simulink model "Acceleration"  (R2017a)
settings: Solver=VariableStepAuto  StartTime=0.0  StopTime=5  FixedStep=0.0001  RelTol=1e-3
values from neighbouring files (symbols this model uses):
  Fz0 = 450*g    (= 4414.5)    [variabeln.m]
  g = 9.81    [variabeln.m]
  gear_ratio = 7.13    [variabeln.m]
  h_CoM = 0.5    [variabeln.m]
  J = 1    [variabeln.m]
  K_i = 100    [variabeln.m]
  l = l_f+l_r    (= 3)    [variabeln.m]
  l_f = 1.5    [variabeln.m]
  lambda_target = 0.1    [variabeln.m]
  m = 700    [variabeln.m]
  max_torque = 220    [variabeln.m]
  Q = 1000    [variabeln.m]
  R = 0.01    [variabeln.m]
  r = 0.25    [variabeln.m]
  Ta0 = 800    [variabeln.m]
  theta1 = 0.86    [variabeln.m]
  theta2 = 33.82    [variabeln.m]
  theta3 = 0.35    [variabeln.m]
  w0 = 200    [variabeln.m]
  W_luft = 0.5*cw*A*rho    (= 0.45)    [variabeln.m]
settings Model: Creator=frede  LastModifiedBy=Dominic
settings DataIOCC: ExternalInput=[t, u,m,g,r,J,theta1,theta2,theta3,v0,gear_ratio,v_max]
settings DebuggingCC: MaxConsecutiveZCsMsg=none

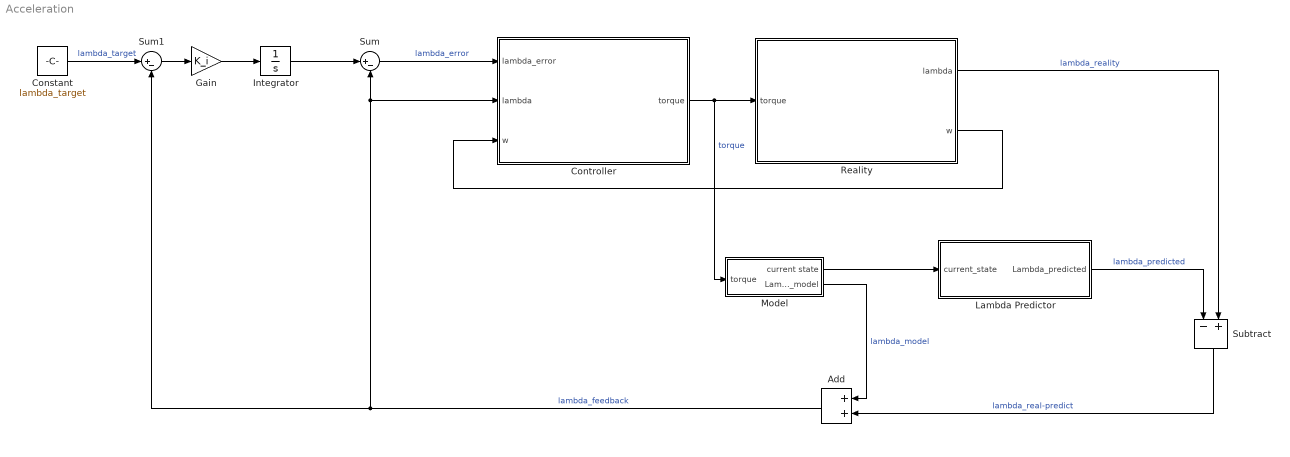
== system Acceleration ==
  Add : Sum
  Constant : Constant  Value=lambda_target
  Controller : Subsystem
  Gain : Gain  Gain=K_i
  Integrator : Integrator
  Lambda Predictor : Subsystem
  Model : Subsystem
  Reality : Subsystem
  Subtract : Sum  Inputs=-+
  Sum : Sum  Inputs=|+-
  Sum1 : Sum  Inputs=|+-
  wires:
  Sum/1 -> Controller/1(lambda_error)  "lambda_error"
  Controller/1(torque) -> Model/1(torque), Reality/1(torque)  "torque"
  Constant/1 -> Sum1/1  "lambda_target"
  Reality/1(lambda) -> Subtract/2  "lambda_reality"
  Sum1/1 -> Gain/1
  Reality/2(w) -> Controller/3(w)
  Integrator/1 -> Sum/1
  Subtract/1 -> Add/2  "lambda_real-predict"
  Model/1(current state) -> Lambda Predictor/1(current_state)
  Lambda Predictor/1(Lambda_predicted) -> Subtract/1  "lambda_predicted"
  Gain/1 -> Integrator/1
  Add/1 -> Controller/2(lambda), Sum/2, Sum1/2  "lambda_feedback"
  Model/2(Lambda_model) -> Add/1  "lambda_model"

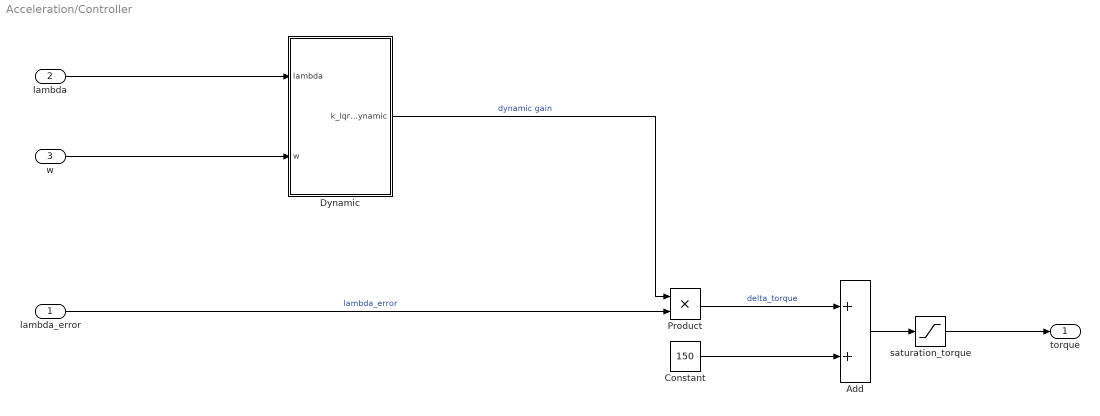
== system Acceleration/Controller ==
  lambda_error : Inport
  lambda : Inport  Port=2
  w : Inport  Port=3
  Add : Sum
  Constant : Constant  Value=150
  Dynamic : MATLAB Function  TreatAsAtomicUnit=on
  Product : Product
  saturation_torque : Saturate  UpperLimit=max_torque  LowerLimit=0
  torque : Outport
  wires:
  Add/1 -> saturation_torque/1
  Product/1 -> Add/1  "delta_torque"
  lambda_error/1 -> Product/2  "lambda_error"
  Constant/1 -> Add/2
  w/1 -> Dynamic/2(w)
  saturation_torque/1 -> torque/1
  Dynamic/1(k_lqr_dynamic) -> Product/1  "dynamic gain"
  lambda/1 -> Dynamic/1(lambda)

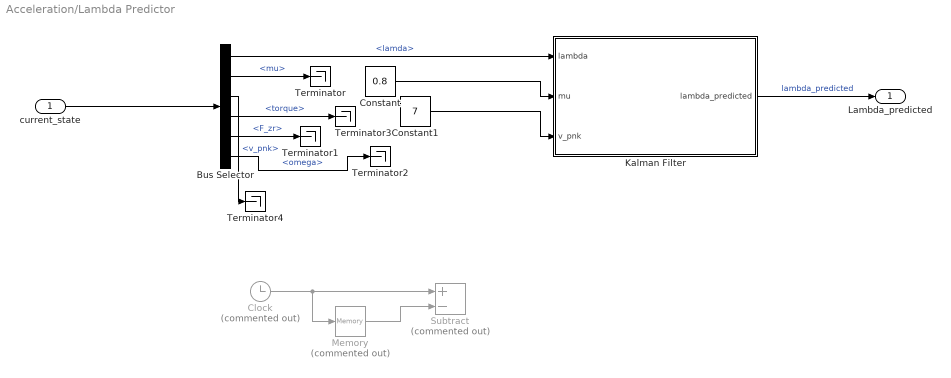
== system Acceleration/Lambda Predictor ==
  current_state : Inport
  Bus Selector : BusSelector  OutputSignals=lamda,mu,v_pnk,torque,F_zr,omega
  Clock : Clock  Commented=on
  Constant : Constant  Value=0.8
  Constant1 : Constant  Value=7
  Kalman Filter : MATLAB Function  TreatAsAtomicUnit=on
  Memory : Memory  Commented=on
  Subtract : Sum  Commented=on  Inputs=+-
  Terminator{,1..4} (5 alike) : Terminator
  Lambda_predicted : Outport
  wires:
  Kalman Filter/1(lambda_predicted) -> Lambda_predicted/1  "lambda_predicted"
  current_state/1 -> Bus Selector/1
  Bus Selector/1 -> Kalman Filter/1(lambda)  "<lamda>"
  Bus Selector/3 -> Terminator4/1  "<v_pnk>"
  Bus Selector/4 -> Terminator3/1  "<torque>"
  Bus Selector/5 -> Terminator1/1  "<F_zr>"
  Bus Selector/2 -> Terminator/1  "<mu>"
  Constant/1 -> Kalman Filter/2(mu)
  Bus Selector/6 -> Terminator2/1  "<omega>"
  Constant1/1 -> Kalman Filter/3(v_pnk)
  Clock/1 -> Memory/1, Subtract/1
  Memory/1 -> Subtract/2

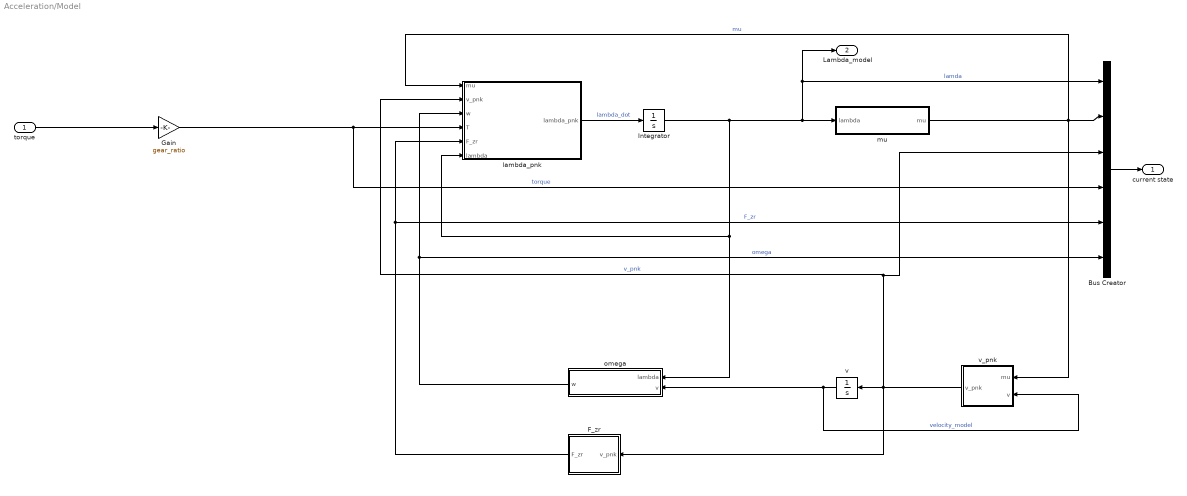
== system Acceleration/Model ==
  torque : Inport
  Bus Creator : BusCreator  Inputs=6
  F_zr : MATLAB Function  TreatAsAtomicUnit=on
  Gain : Gain  Gain=gear_ratio
  Integrator : Integrator
  lambda_pnk : MATLAB Function  TreatAsAtomicUnit=on
  mu : MATLAB Function  TreatAsAtomicUnit=on
  omega : MATLAB Function  TreatAsAtomicUnit=on
  v : Integrator  InitialCondition=0.1
  v_pnk : MATLAB Function  TreatAsAtomicUnit=on
  current state : Outport
  Lambda_model : Outport  Port=2
  wires:
  Integrator/1 -> omega/1(lambda), lambda_pnk/6(lambda), Lambda_model/1, Bus Creator/1, mu/1(lambda)  "lamda"
  mu/1(mu) -> Bus Creator/2, v_pnk/1(mu), lambda_pnk/1(mu)  "mu"
  v_pnk/1(v_pnk) -> Bus Creator/3, lambda_pnk/2(v_pnk), v/1, F_zr/1(v_pnk)  "v_pnk"
  F_zr/1(F_zr) -> Bus Creator/5, lambda_pnk/5(F_zr)  "F_zr"
  lambda_pnk/1(lambda_pnk) -> Integrator/1  "lambda_dot"
  omega/1(w) -> Bus Creator/6, lambda_pnk/3(w)  "omega"
  v/1 -> omega/2(v), v_pnk/2(v)  "velocity_model"
  torque/1 -> Gain/1
  Gain/1 -> Bus Creator/4, lambda_pnk/4(T)  "torque"
  Bus Creator/1 -> current state/1

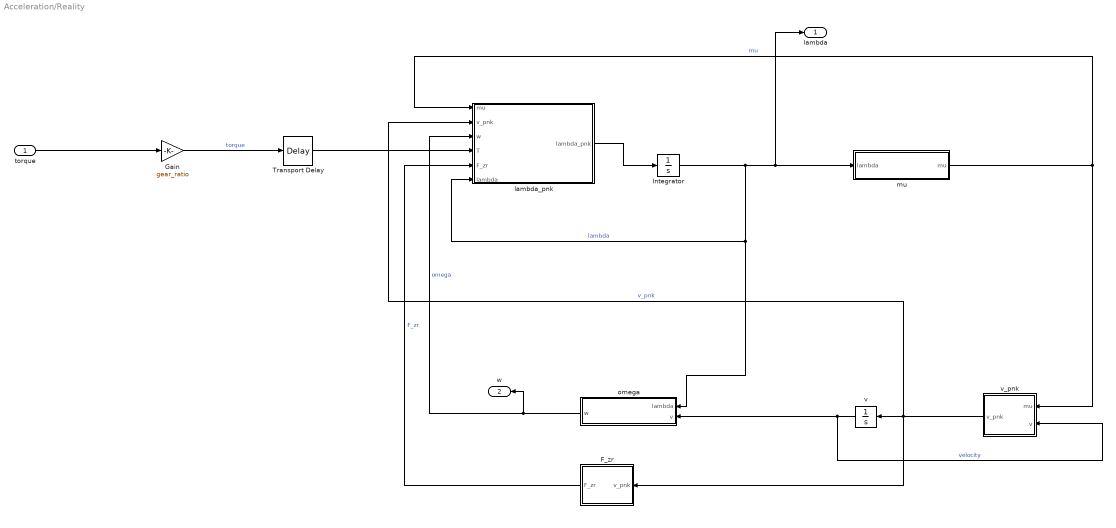
== system Acceleration/Reality ==
  torque : Inport
  F_zr : MATLAB Function  TreatAsAtomicUnit=on
  Gain : Gain  Gain=gear_ratio
  Integrator : Integrator
  Transport Delay : TransportDelay  DelayTime=0.2
  lambda_pnk : MATLAB Function  TreatAsAtomicUnit=on
  mu : MATLAB Function  TreatAsAtomicUnit=on
  omega : MATLAB Function  TreatAsAtomicUnit=on
  v : Integrator  InitialCondition=0.1
  v_pnk : MATLAB Function  TreatAsAtomicUnit=on
  lambda : Outport
  w : Outport  Port=2
  wires:
  Integrator/1 -> omega/1(lambda), lambda_pnk/6(lambda), lambda/1, mu/1(lambda)  "lambda"
  mu/1(mu) -> lambda_pnk/1(mu), v_pnk/1(mu)  "mu"
  v_pnk/1(v_pnk) -> lambda_pnk/2(v_pnk), v/1, F_zr/1(v_pnk)  "v_pnk"
  F_zr/1(F_zr) -> lambda_pnk/5(F_zr)  "F_zr"
  lambda_pnk/1(lambda_pnk) -> Integrator/1
  omega/1(w) -> w/1, lambda_pnk/3(w)  "omega"
  v/1 -> omega/2(v), v_pnk/2(v)  "velocity"
  torque/1 -> Gain/1
  Gain/1 -> Transport Delay/1  "torque"
  Transport Delay/1 -> lambda_pnk/4(T)

== matlab function Acceleration/Reality/mu ==
  data: lambda input; mu output; theta1 parameter; theta2 parameter; theta3 parameter
function mu = mu(lambda, theta1, theta2, theta3)

if lambda>=0
    mu = theta1*(1-exp(-theta2*lambda))-lambda*theta3;
    
else
         mu = -(theta1*(1-exp(-theta2*abs(lambda)))-abs(lambda)*theta3);


end

== matlab function Acceleration/Lambda Predictor/Kalman Filter ==
  data: lambda input; mu input; lambda_predicted output; v_pnk input; r parameter; J parameter; Ta0 parameter; Fz0 parameter; w0 parameter
function lambda_predicted = fcn(lambda,mu,v_pnk,r,J,Ta0,Fz0, w0)



%% Initial State

F=-v_pnk/(w0*r)+(1-lambda)/w0*Ta0/J-(1-lambda)/w0*r*Fz0*mu/J;

time = 0.01;
%% Initializing
nSteps = 0.2/time;
L=zeros(1,nSteps);
L(1)=lambda;


%% Predicting
for k = 2:nSteps
     L(k)= L(k-1) + F*time;
end
     
lambda_predicted = L(nSteps);


end

== matlab function Acceleration/Reality/F_zr ==
  data: F_zr output; v_pnk input; m parameter; h_CoM parameter; l parameter; g parameter; l_f parameter
function F_zr = fcn(v_pnk,m, h_CoM, l, g, l_f)

F_zr=m*h_CoM/l*v_pnk+m*g*l_f/l;

end

== matlab function Acceleration/Reality/lambda_pnk ==
  data: mu input; v_pnk input; lambda_pnk output; w input; T input; F_zr input; r parameter; J parameter; lambda input
function lambda_pnk = fcn(mu,v_pnk,w,T,F_zr, r, J,lambda)

lambda_pnk=-v_pnk/(w*r)+(1-lambda)/w*T/J-(1-lambda)/w*r*F_zr*mu/J;

end

== matlab function Acceleration/Reality/omega ==
  data: lambda input; v input; w output; r parameter
function w = fcn(lambda, v,r)

w=v/(1-lambda)/r;

end

== matlab function Acceleration/Reality/v_pnk ==
  data: mu input; v_pnk output; g parameter; l_f parameter; l parameter; h_CoM parameter; v input; W_luft parameter; m parameter
function v_pnk = fcn(mu,g, l_f, l, h_CoM,v,W_luft, m)

v_pnk=mu*g*l_f/(l-mu*h_CoM)-W_luft/((1-h_CoM/l*mu)*m)*v^2;

end

== matlab function Acceleration/Model/F_zr ==
  data: F_zr output; v_pnk input; m parameter; h_CoM parameter; l parameter; g parameter; l_f parameter
function F_zr = fcn(v_pnk,m, h_CoM, l, g, l_f)

F_zr=m*h_CoM/l*v_pnk+m*g*l_f/l;

end

== matlab function Acceleration/Controller/Dynamic ==
  data: lambda input; k_lqr_dynamic output; w input; m parameter; r parameter; J parameter; theta1 parameter; theta2 parameter; theta3 parameter; R parameter; Q parameter; Fz0 parameter; Ta0 parameter
function k_lqr_dynamic = fcn(lambda, w,m, r, J, theta1, theta2, theta3, R, Q, Fz0, Ta0)



A1=Ta0/(J*w)-Fz0*r/(J*w)*(theta1*theta2*exp(-lambda*theta2)-theta3)+Fz0*r/(J*w)* ...
    (theta1*(1-exp(-lambda*theta2)-lambda*theta2*exp(-lambda*theta2))-2*lambda*theta3) ...
    -Fz0/(m*r*w)*(theta1*theta2*exp(-lambda*theta2)-theta3);

B1=1/(J*w)-lambda/(J*w);


    k_lqr_dynamic =(A1+B1*sqrt(A1^2+B1^2*Q/R))/B1;

end

== matlab function Acceleration/Model/lambda_pnk ==
  data: mu input; v_pnk input; lambda_pnk output; w input; T input; F_zr input; r parameter; J parameter; lambda input
function lambda_pnk = fcn(mu,v_pnk,w,T,F_zr, r, J,lambda)

lambda_pnk=-v_pnk/(w*r)+(1-lambda)/w*T/J-(1-lambda)/w*r*F_zr*mu/J;

end

== matlab function Acceleration/Model/mu ==
  data: lambda input; mu output; theta1 parameter; theta2 parameter; theta3 parameter
function mu = mu(lambda, theta1, theta2, theta3)

if lambda>=0
    mu = theta1*(1-exp(-theta2*lambda))-lambda*theta3;
    
else
         mu = -(theta1*(1-exp(-theta2*abs(lambda)))-abs(lambda)*theta3);


end

== matlab function Acceleration/Model/omega ==
  data: lambda input; v input; w output; r parameter
function w = fcn(lambda, v,r)

w=v/(1-lambda)/r;

end

== matlab function Acceleration/Model/v_pnk ==
  data: mu input; v_pnk output; g parameter; l_f parameter; l parameter; h_CoM parameter; v input; W_luft parameter; m parameter
function v_pnk = fcn(mu,g, l_f, l, h_CoM,v,W_luft, m)

v_pnk=mu*g*l_f/(l-mu*h_CoM)-W_luft/((1-h_CoM/l*mu)*m)*v^2;

end
